simulink model "sl_drivepose_vs"  (R2015b)
settings: Solver=ode45  StartTime=0.0  StopTime=10  MaxStep=0.05  RelTol=1e-3
InitFcn:
  | camera = CentralCamera('default', 'focal', 0.002);
  | P = [4 10 3; 9 9 2; 6 8 3; 8 10 4; 10 7 2]';
  | T_VC = transl(0.2, 0.1, 0.5)*troty(pi/2)*trotz(-pi/2);
  | x0 = [2 2 0];
  | xg = [5 5 pi/2];
libraries: roblocks x9, simulink x1
settings Model: Creator=pic  LastModifiedBy=corkep
settings DataIOCC: LimitDataPoints=off  SaveFormat=Array  SignalLoggingSaveFormat=ModelDataLogs  SaveState=on  ReturnWorkspaceOutputs=on
settings OptimizationCC: ExpressionDepthLimit=2147483647
settings DebuggingCC: UnderspecifiedInitializationDetection=Classic  MergeDetectMultiDrivingBlocksExec=none  SolverPrmCheckMsg=warning  FcnCallInpInsideContextMsg=UseLocalSettings  StateNameClashWarn=warning
settings HardwareCC: ProdBitPerPointer=32  ProdLargestAtomicFloat=None  ProdIntDivRoundTo=Undefined  ProdEndianess=Unspecified  ProdWordSize=32  ProdHWDeviceType=32-bit Generic
settings GRTTargetCC: GeneratePreprocessorConditionals=Disable all  CombineOutputUpdateFcns=off  GRTInterface=on
settings ConfigComp: CovModelRefEnable=Off  CovSFcnEnable=off

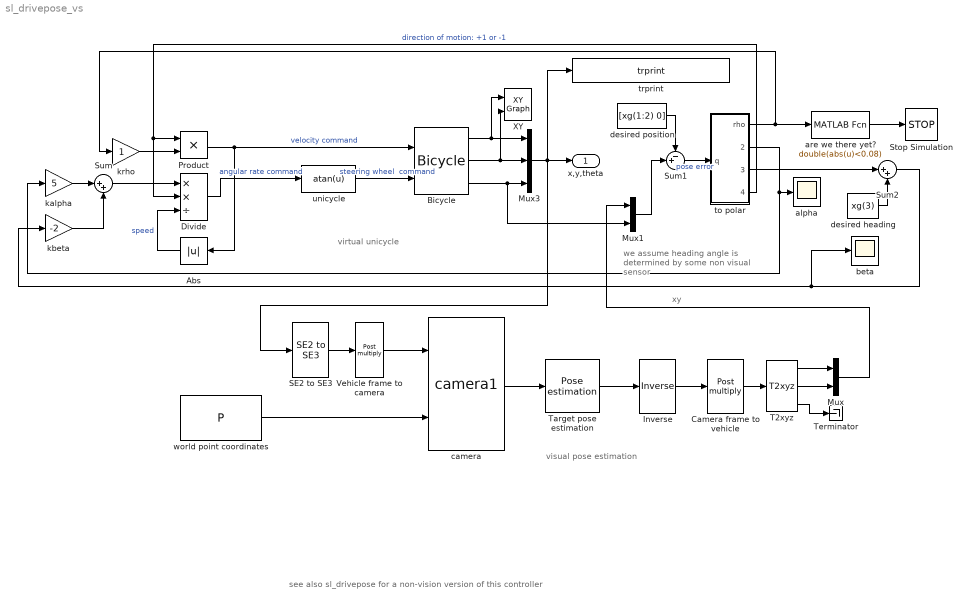
== system sl_drivepose_vs ==
  note: we assume heading angle
      | is determined by some non visual sensor
  note: visual pose estimation
  note: see also sl_drivepose for a non-vision version of this controller
  note: xy
  note: virtual unicycle
  Abs : Abs
  Bicycle : roblocks/Vehicles/Bicycle  vlim=1  accel=1  alim=1  steer_rate=Inf  L=1  x0=x0
  Camera frame to vehicle : roblocks/Toolbox/Post multiply  T2=inv(T_VC)
  Divide : Product  Inputs=**/
  Inverse : roblocks/Toolbox/Inverse
  Mux : Mux  Inputs=2
  Mux1 : Mux  Inputs=2
  Mux3 : Mux  Inputs=3
  Product : Product  RndMeth=Zero
  SE2 to SE3 : roblocks/Toolbox/SE2 to SE3
  Stop Simulation : Stop
  Sum : Sum  Inputs=|++
  Sum1 : Sum  Inputs=-+|
  Sum2 : Sum  Inputs=|++
  T2xyz : roblocks/Toolbox/T2xyz
  Target pose estimation : roblocks/Vision/Pose estimation  cam=camera  P=P
  Terminator : Terminator
  Vehicle frame to camera : roblocks/Toolbox/Post multiply  T2=T_vc
  XY : simulink/Sinks/XY Graph  xmin=0  xmax=10  ymin=0  ymax=10  st=-1
  alpha : Scope
  are we there yet? : MATLABFcn  MATLABFcn=double(abs(u)<0.08)  OutputSignalType=real
  beta : Scope
  camera : roblocks/Vision/camera1  cam=camera
  desired heading : Constant  Value=xg(3)
  desired position : Constant  Value=[xg(1:2) 0]
  kalpha : Gain  Gain=5
  kbeta : Gain  Gain=-2
  krho : Gain
  to polar : Subsystem
  trprint : roblocks/Toolbox/trprint  options={}
      link override S-Function: Parameters=options
  "unicycle " : Fcn  Expr=atan(u)
  world point coordinates : Constant  Value=P  VectorParams1D=off
  x,y,theta : Outport
  wires:
  Mux3/1 -> trprint/1, SE2 to SE3/1, x,y,theta/1
  Bicycle/1 -> Mux3/1, XY/1
  Bicycle/2 -> Mux3/2, XY/2
  Bicycle/3 -> Mux1/2, Mux3/3
  to polar/2(alpha) -> kalpha/1, alpha/1
  kalpha/1 -> Sum/1
  kbeta/1 -> Sum/2
  Product/1 -> Bicycle/1, Abs/1  "velocity command"
  krho/1 -> Product/2
  to polar/1(rho) -> are we there yet?/1, krho/1
  to polar/4(direction) -> Product/1, Divide/2  "direction of motion: +1 or -1"
  desired position/1 -> Sum1/1
  Sum1/1 -> to polar/1(q)  "pose error"
  Sum/1 -> Divide/1
  are we there yet?/1 -> Stop Simulation/1
  to polar/3(beta) -> Sum2/1
  Sum2/1 -> kbeta/1, beta/1
  desired heading/1 -> Sum2/2
  Divide/1 -> "unicycle "/1  "angular rate command"
  Abs/1 -> Divide/3  "speed"
  "unicycle "/1 -> Bicycle/2  "steering wheel  command"
  Vehicle frame to camera/1 -> camera/1
  SE2 to SE3/1 -> Vehicle frame to camera/1
  Target pose estimation/1 -> Inverse/1
  Camera frame to vehicle/1 -> T2xyz/1
  Inverse/1 -> Camera frame to vehicle/1
  world point coordinates/1 -> camera/2
  camera/1 -> Target pose estimation/1
  T2xyz/1 -> Mux/1
  T2xyz/2 -> Mux/2
  Mux/1 -> Mux1/1
  Mux1/1 -> Sum1/2
  T2xyz/3 -> Terminator/1

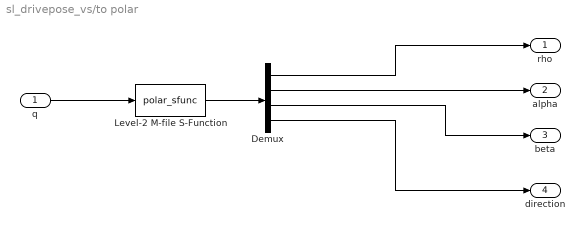
== system sl_drivepose_vs/to polar ==
  q : Inport
  Demux : Demux
  Level-2 M-file S-Function : M-S-Function  FunctionName=polar_sfunc
  rho : Outport
  alpha : Outport  Port=2
  beta : Outport  Port=3
  direction : Outport  Port=4
  wires:
  Demux/3 -> beta/1
  q/1 -> Level-2 M-file S-Function/1
  Level-2 M-file S-Function/1 -> Demux/1
  Demux/1 -> rho/1
  Demux/2 -> alpha/1
  Demux/4 -> direction/1
